simulink model "SProfilePlan_code"  (R2022a)
settings: Solver=FixedStepDiscrete  StartTime=0.0  StopTime=10.0  FixedStep=0.001  RelTol=1e-3  EnableMultiTasking=on
settings Model: Creator=randolf  LastModifiedBy=randolf
settings SolverCC: AlgebraicLoopSolver=TrustRegion  AutoInsertRateTranBlk=on
settings DataIOCC: LimitDataPoints=on
settings OptimizationCC: LifeSpan=inf
settings DebuggingCC: UnconnectedInputMsg=warning  UnconnectedOutputMsg=warning  UnconnectedLineMsg=warning  AllowSymbolicDim=off  SFUnexpectedBacktrackingDiag=warning  SFNoUnconditionalDefaultTransitionDiag=warning  SFExecutionAtInitializationDiag=none  ArithmeticOperatorsInVariantConditions=warning
settings SFSimCC: SimUseLocalCustomCode=off  CustomCodeUndefinedFunction=UseInterfaceOnly
settings RTWCC: RTWUseLocalCustomCode=off  DLArmComputeVersion=19.05
settings CodeAppCC: StateflowObjectComments=on
settings GRTTargetCC: TargetLangStandard=C89/C90 (ANSI)
settings ConfigComp: CovMetricSettings=dw  CovSaveCumulativeToWorkspaceVar=on  CovSaveSingleToWorkspaceVar=on  CovExternalEMLEnable=off  CovSFcnEnable=off

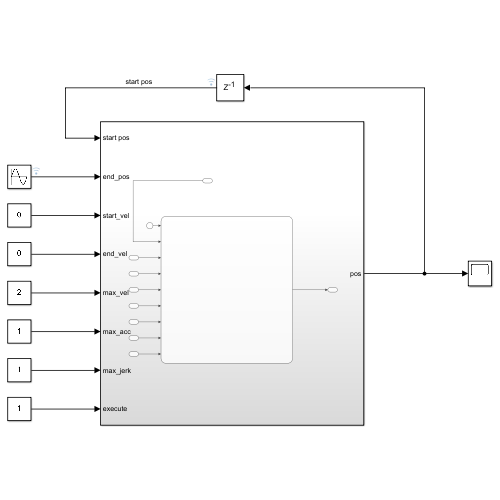
[thumbnail: Simulink's stored preview of the top-level diagram]
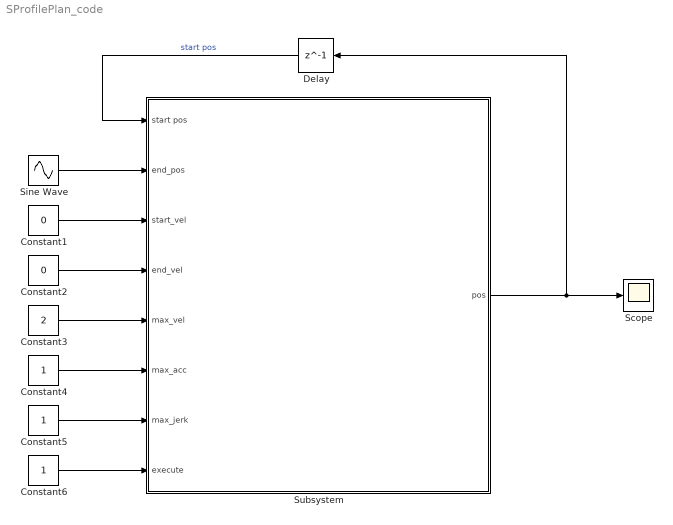
== system SProfilePlan_code ==
  Constant1 : Constant  Value=0
  Constant2 : Constant  Value=0
  Constant3 : Constant  Value=2
  Constant4 : Constant
  Constant5 : Constant
  Constant6 : Constant
  Delay : Delay  DelayLength=1
  Scope : Scope
  Sine Wave : Sin  SampleTime=0
  Subsystem : Subsystem
  wires:
  Subsystem/1(pos) -> Scope/1, Delay/1
  Delay/1 -> Subsystem/1(start pos)  "start pos"
  Sine Wave/1 -> Subsystem/2(end_pos)
  Constant1/1 -> Subsystem/3(start_vel)
  Constant2/1 -> Subsystem/4(end_vel)
  Constant3/1 -> Subsystem/5(max_vel)
  Constant4/1 -> Subsystem/6(max_acc)
  Constant5/1 -> Subsystem/7(max_jerk)
  Constant6/1 -> Subsystem/8(execute)

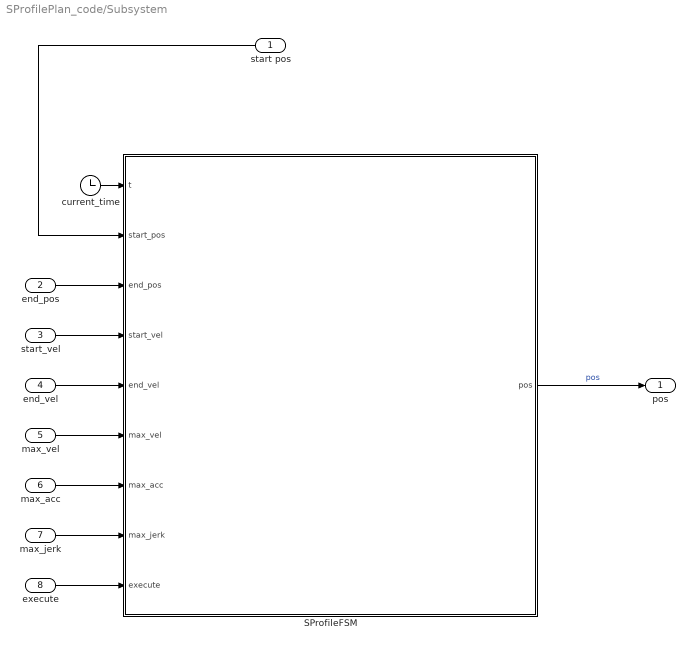
== system SProfilePlan_code/Subsystem ==
  start pos : Inport
  end_pos : Inport  Port=2
  start_vel : Inport  Port=3
  end_vel : Inport  Port=4
  max_vel : Inport  Port=5
  max_acc : Inport  Port=6
  max_jerk : Inport  Port=7
  execute : Inport  Port=8
  SProfileFSM : Stateflow chart  TreatAsAtomicUnit=on
  current_time : Clock
  pos : Outport
  wires:
  SProfileFSM/1(pos) -> pos/1  "pos"
  current_time/1 -> SProfileFSM/1(t)
  end_pos/1 -> SProfileFSM/3(end_pos)
  execute/1 -> SProfileFSM/9(execute)
  start_vel/1 -> SProfileFSM/4(start_vel)
  max_jerk/1 -> SProfileFSM/8(max_jerk)
  end_vel/1 -> SProfileFSM/5(end_vel)
  max_vel/1 -> SProfileFSM/6(max_vel)
  max_acc/1 -> SProfileFSM/7(max_acc)
  start pos/1 -> SProfileFSM/2(start_pos)

== stateflow chart SProfilePlan_code/Subsystem/SProfileFSM ==
  state HoldOn
    entry:
    T = 5;
    current_pos = start_pos;
    during:
    pos = current_pos;
  state InitParam
    entry:
    start_t = t;
    param = zeros(1,16);
    sigma = sign(end_pos - start_pos);
    param = STrajectoryPara(start_pos, end_pos, start_vel, end_vel, max_vel, max_acc, max_jerk);
    T = param(1) + param(2) + param(3);
  state GeneratePos
    during:
    if (t-start_t) <= T
    pos = sigma * S_position(t-start_t, param(1), param(2), param(3), param(4), param(5), param(6), param(7), param(8), param(9), param(10), param(11), param(12), param(13), param(14), param(15), param(16));
    else
    pos = end_pos;
    end
    current_pos = pos;
  (default) -> HoldOn
  GeneratePos -> HoldOn : [(t-start_t)>T]
  HoldOn -> InitParam : [execute==1 && abs(end_pos-start_pos)>1e-4]
  InitParam -> GeneratePos : [true]
  data: t input; start_pos input; end_pos input; start_vel input; end_vel input; max_vel input; max_acc input; max_jerk input; execute input; T local size=1; sigma local size=1; param local size=1, 16; pos output size=1; current_pos local; start_t local
